simulink model "QPSKMODEM"  (R2020b)
settings: Solver=VariableStepAuto  StartTime=0.0  StopTime=inf  RelTol=1e-3
model workspace (MAT data in the model file):
  BitRate = 20480
  CoreFreq = 40960
  RCF_Rolloff_factor = 0.1
  SampleRateQPSK = 819200
undefined symbols (not defined in the file): fdesignblkfcn, gcbh, random
libraries: simulink_extras x9, simulink x6, commfilt2 x4, dspsrcs4 x3, commrfcorlib x2, commutil2 x2, dspmathops x2, commrandsrc3 x1, commsink2 x1, commchan3 x1
(part 2 of 2)

== system QPSKMODEM/Reciever/Symbol_clk_restorator/Bandpass Filter2 ==
  In : Inport
  Generated Filter Block : DiscreteFir  Tag=BlockMethodSubSystem  Coefficients=[1.33291293613741489e-06 -3.71729674503269073e-06 -2.55982433042465191e-06 -2.3244966415084971e-06 -2.0722245476230491e-06 -1.50854830451986809e-06 -5.72891685133694265e-07 6.65656947025783295e-07 2.04911167673330056e-06 3.35197704869231731e-06 4.32055999851877012e-06 4.71151414744170765e-06 4.34530519577557304e-06 3.14564616485739826e-06 1.17753788969815406e-06 -1.34636792999603235e-06 -4.07375681599398936e-06 -6.56025667124246123e-06 -8.32830846950749775e-06 -8.95475221998336354e-06 -8.14768533239771636e-06 -5.8259593796378098e-06 -2.15690289505963077e-06 2.42768022547142276e-06 7.27866172757355486e-06 1.16014189686021614e-05 1.4586450061584313e-05 1.55339848578051398e-05 1.40086871319831641e-05 9.92697107453206786e-06 3.64974736138616162e-06 -4.0649354262165857e-06 -1.20930363766651291e-05 -1.91304462997007023e-05 -2.38835268125860489e-05 -2.52595024430426598e-05 -2.26226286098086369e-05 -1.59322907835080267e-05 -5.8230715145782389e-06 6.42819751348861043e-06 1.90338354835750395e-05 2.99458667561533163e-05 3.71668264264164933e-05 3.90947632637926118e-05 3.48304656309026539e-05 2.44069925721513521e-05 8.88074976814050208e-06 -9.73414589850726173e-06 -2.8703505146679707e-05 -4.49514345798067013e-05 -5.55378556077206398e-05 -5.81583294413739419e-05 -5.15899573692238451e-05 -3.59995863972453691e-05 -1.30518143912198537e-05 1.42212426546720768e-05 4.17898549903912732e-05 6.5194728062666646e-05 8.02417564023146776e-05 8.37132768455236273e-05 7.39872746307630041e-05 5.14473521720787956e-05 1.85967920979521701e-05 -2.01545172868308598e-05 -5.90584458982579085e-05 -9.18331833531083172e-05 -0.000112657573781342699 -0.000117152435651038335 -0.000103214617718458597 -7.15506955373990968e-05 -2.57990541768897453e-05 2.78269231657254816e-05 8.13363112470276986e-05 0.0001261150273754031 0.000154270437507517491 0.000159970002534428777 0.00014054476822755396 9.71680622123971961e-05 3.49586967850069982e-05 -3.7543941000230478e-05 -0.000109502657605406337 -0.00016935774900787799 -0.000206639206936389138 -0.000213732395340630627 -0.000187313692288571508 -0.000129193034557493038 -4.6391288403871765e-05 4.96216147612247059e-05 0.000144455257338812571 0.000222909604845972491 0.000271354986875024426 0.000280031031321154467 0.000244867170379394253 0.000168524530020135638 6.0410638870396045e-05 -6.43757209733221333e-05 -0.000187090084176245834 -0.000288104887231354051 -0.000349987496540658588 -0.000360426665037735664 -0.000314524064490422387 -0.000216037916425287387 -7.73228293229287196e-05 8.21099480516207248e-05 0.000238265479255448081 0.000366218525796791925 0.000444025874211647319 0.000456397849892745469 0.000397523992669530988 0.000272553928949029168 9.74142095137955536e-05 -0.000103101460023173242 -0.000298765733713606246 -0.000458409264960771593 -0.000554817290313541853 -0.000569267289588973389 -0.000494969698399205056 -0.000338796460210581977 -0.000120935877677477211 0.000127591262896608324 0.00036926412578416754 0.000565661311626165808 0.000683492929052940327 0.000700137004399498759 0.000607768671461196282 0.000415354283618889816 0.000148089637033452096 -0.000155766743255090394 -0.000450282512722346225 -0.000688725149942851053 -0.000830901168858613607 -0.000849816758113741688 -0.000736574061871812509 -0.000502642351229692116 -0.000179016349192079923 0.000187749991531884695 0.000542151484787903228 0.000828060744966827196 0.000997539170306453379 0.00101875684840367522 0.000881728783528820843 0.000600863951675842172 0.000213781511948922374 -0.000223583327422953622 -0.000644974405495246737 -0.000983780922026523128 -0.00118348871639559401 -0.001206986428611575 -0.00104321153086955323 -0.000709975363607827934 -0.000252363502226554475 0.00026321835999364477 0.000758594950399557252 0.00115560522993273245 0.00138836042753224349 0.00141405651139719316 0.00122059160224736009 0.000829656527376232324 0.000294642223916765896 -0.000306507808665003583 -0.000882570147217811782 -0.00134282083196826229 -0.00161125044688458646 -0.0016389999409642073 ...(+10366 chars)]
  Out : Outport  VectorParamsAs1DForOutWhenUnconnected=off
  wires:
  In/1 -> Generated Filter Block/1
  Generated Filter Block/1 -> Out/1

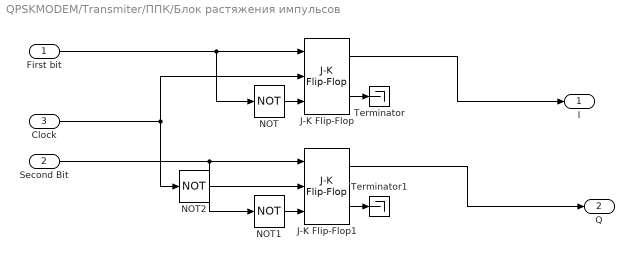
== system QPSKMODEM/Transmiter/ППК/Блок растяжения импульсов ==
  First bit : Inport
  Second Bit : Inport  Port=2
  Clock : Inport  Port=3
  J-K Flip-Flop : simulink_extras/Flip Flops/J-K Flip-Flop  initial_condition=0
  J-K Flip-Flop1 : simulink_extras/Flip Flops/J-K Flip-Flop  initial_condition=0
  NOT : Logic  Operator=NOT  IconShape=distinctive  AllPortsSameDT=off  OutDataTypeStr=boolean
  NOT1 : Logic  Operator=NOT  IconShape=distinctive  AllPortsSameDT=off  OutDataTypeStr=boolean
  NOT2 : Logic  Operator=NOT  IconShape=distinctive  AllPortsSameDT=off  OutDataTypeStr=boolean
  Terminator : Terminator
  Terminator1 : Terminator
  I : Outport  VectorParamsAs1DForOutWhenUnconnected=off
  Q : Outport  Port=2  VectorParamsAs1DForOutWhenUnconnected=off
  wires:
  First bit/1 -> NOT/1, J-K Flip-Flop/1
  NOT/1 -> J-K Flip-Flop/3
  NOT1/1 -> J-K Flip-Flop1/3
  Second Bit/1 -> NOT1/1, J-K Flip-Flop1/1
  J-K Flip-Flop/1 -> I/1
  J-K Flip-Flop1/1 -> Q/1
  Clock/1 -> J-K Flip-Flop/2, NOT2/1
  NOT2/1 -> J-K Flip-Flop1/2
  J-K Flip-Flop/2 -> Terminator/1
  J-K Flip-Flop1/2 -> Terminator1/1

== system QPSKMODEM/Transmiter/ППК/Демультиплексор ==
  D : Inport
  Code : Inport  Port=2
  Logical Operator : Logic  AllPortsSameDT=off  OutDataTypeStr=boolean
  Logical Operator1 : Logic  AllPortsSameDT=off  OutDataTypeStr=boolean
  Logical Operator2 : Logic  Operator=NOT  AllPortsSameDT=off  OutDataTypeStr=boolean
  A1 : Outport  VectorParamsAs1DForOutWhenUnconnected=off
  A2 : Outport  Port=2  VectorParamsAs1DForOutWhenUnconnected=off
  wires:
  Code/1 -> Logical Operator1/2, Logical Operator2/1
  D/1 -> Logical Operator/1, Logical Operator1/1
  Logical Operator/1 -> A2/1
  Logical Operator1/1 -> A1/1
  Logical Operator2/1 -> Logical Operator/2
